simulink model "mcp23017_task"  (Simulink 7.5)
libraries: mathlib x8, logiclib x2, speclib x1
settings Model: Creator=jsobota  LastModifiedBy=jsobota  ExtModeTrigMode=oneshot  ExtModeArmWhenConnect=off

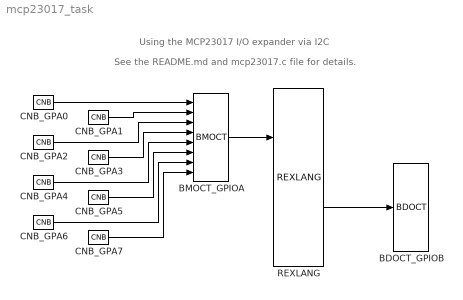
== system mcp23017_task ==
  note: Using the MCP23017 I/O expander via I2C
  note: See the README.md and mcp23017.c file for details.
  BDOCT_GPIOB : logiclib/BDOCT  shift=0
  BMOCT_GPIOA : logiclib/BMOCT  shift=0
  CNB_GPA{0,2,4,6} (4 alike) : mathlib/CNB  YCN=off
  CNB_GPA{1,3,5,7} (4 alike) : mathlib/CNB  YCN=on
  REXLANG : speclib/REXLANG  SystemSampleTime=-1  tab_matlab=BASIC  srcname=mcp23017.c  srctype=1: STL  stack=0  debug=1: No check  p0=0  p1=0  p2=0  p3=0  p4=0  p5=0  p6=0  p7=0  p8=0  p9=0  p10=0  p11=0  p12=0  p13=0  p14=0  p15=0  fname=/dev/i2c-1
  wires:
  BMOCT_GPIOA/1 -> REXLANG/5
  CNB_GPA0/1 -> BMOCT_GPIOA/1
  CNB_GPA1/1 -> BMOCT_GPIOA/2
  CNB_GPA2/1 -> BMOCT_GPIOA/3
  CNB_GPA3/1 -> BMOCT_GPIOA/4
  CNB_GPA4/1 -> BMOCT_GPIOA/5
  CNB_GPA5/1 -> BMOCT_GPIOA/6
  CNB_GPA6/1 -> BMOCT_GPIOA/7
  CNB_GPA7/1 -> BMOCT_GPIOA/8
  REXLANG/12 -> BDOCT_GPIOB/1
